simulink subsystem "PvtSubSys_LONC"  (R2020b)
settings: Solver=VariableStepAuto  StartTime=0.0  StopTime=10.0  RelTol=1e-3
undefined symbols (not defined in the file): P_Global_TireRadius_m, P_Global_Weight_N, P_LongCtrl_AxvRoadSlopeThrd, P_LongCtrl_SlideFlagEnable, P_LongCtrl_TotWheelTrqRatio, P_LongCtrl_VLC_fRollCoef, P_LongCtrl_VLC_WindArea, P_LongCtrl_VLCaccelMinHoldXAxis, P_LongCtrl_VLCaccelMinHoldYAxis, P_LongCtrl_VLCaccelMinSlidHoldXAxis, P_LongCtrl_VLCaccelMinSlidHoldYAxis, P_LongCtrl_VLCaDiffCharCoefKiEnableXAxis, P_LongCtrl_VLCaDiffCharCoefKiXAxis, P_LongCtrl_VLCaDtThresUpdateTorq, P_LongCtrl_VLCaXCDeadZoneProp_Y, P_LongCtrl_VLCaxCtrlDevDeadZoneChar_Y, P_LongCtrl_VLCaxCtrlDevEC2DCMax, P_LongCtrl_VLCaxCtrlDevFastQuitDCMode, P_LongCtrl_VLCaxCtrlDevThresAddEC2DCCharYAxis, P_LongCtrl_VLCaxCtrlDevTresAddDC2ECYAxis, P_LongCtrl_VLCaxDtCharAxCtrlDevTresAddDC2ECXAxis, P_LongCtrl_VLCaxDtCharAxCtrlDevTresAddEC2DCXAxis, P_LongCtrl_VLCAxTarDtThreEnableI, P_LongCtrl_VLCaxvRoadSlopeDC4CharXAxis, P_LongCtrl_VLCaxvRoadSlopeDC4CharYAxis, P_LongCtrl_VLCAxvTracMinDC1FullFillXAxis, P_LongCtrl_VLCAxvTracMinDC1FullFillYAxis, P_LongCtrl_VLCcoefFXAxis, P_LongCtrl_VLCcoefFYAxis, P_LongCtrl_VLCcoefIFadeOut1Calc, P_LongCtrl_VLCcoefIFadeOut1Condition, P_LongCtrl_VLCcoefIFadeOut2Calc, P_LongCtrl_VLCcoefIFadeOut2Condition, P_LongCtrl_VLCcoefIFadeOut3Calc, P_LongCtrl_VLCcoefIFadeOut3Condition, P_LongCtrl_VLCcoefKiDiffDtEnlargeYAxis, P_LongCtrl_VLCcoefKiEnableYAxis, P_LongCtrl_VLCcoefKiEnlargeADiffYAxis, P_LongCtrl_VLCcoefPIYAxis, P_LongCtrl_VLCCounterAxvTracMinTimeout, P_LongCtrl_VLCCounterDC2ECTorqDelay, P_LongCtrl_VLCCounterDrvOff2EC, P_LongCtrl_VLCdaxTarEC2DCMax, P_LongCtrl_VLCdiffDtCharCoefKiEnlargeXAxis, P_LongCtrl_VLCdriveOffAxUpLimXAxix, P_LongCtrl_VLCdriveOffAxUpLimYAxix, P_LongCtrl_VLCDtAxvRef2UpperBandDC5, P_LongCtrl_VLCengEfficientCharYAxis, P_LongCtrl_VLCengInverseEfficientYAxis, P_LongCtrl_VLCIACompensionNeg, P_LongCtrl_VLCIACompensionPos, P_LongCtrl_VLCjerkHoldXAxis, P_LongCtrl_VLCjerkHoldYAxis, P_LongCtrl_VLCjerkSlidHoldXAxis, P_LongCtrl_VLCjerkSlidHoldYAxis, P_LongCtrl_VLCki, P_LongCtrl_VLCkp, P_LongCtrl_VLCks, P_LongCtrl_VLCLowerJerkCounterDrvOff2EC, P_LongCtrl_VLCMaRatioCharMaYAxis ... (+12)
libraries: simulink x34
(part 3 of 3)

== matlab function PvtSubSys_LONC/VLC/Vlc/PI_Control/MATLAB Function ==
  data: I_k1 input single; Err input single; ECenable input boolean; I output single; Limited output single; axvFilt output single; Diff input single; tCycle input single; P_VlcWindupLim input single; AxTarDt input single; axv input single; tConst input single; VlcAxTar input single; ShiftInProgress input boolean; axvFiltK1 input single; P_LongCtrl_VLCAxTarDtThreEnableI parameter single; P_LongCtrl_VLCcoefIFadeOut1Condition parameter single; P_LongCtrl_VLCcoefIFadeOut1Calc parameter single; P_LongCtrl_VLCcoefIFadeOut2Condition parameter single; P_LongCtrl_VLCcoefIFadeOut2Calc parameter single; P_LongCtrl_VLCcoefIFadeOut3Condition parameter single; P_LongCtrl_VLCcoefIFadeOut3Calc parameter single; P_LongCtrl_VLCIACompensionPos parameter single; P_LongCtrl_VLCIACompensionNeg parameter single
function [I,Limited,axvFilt] = calcI(I_k1,Err,ECenable,Diff,tCycle,P_VlcWindupLim,AxTarDt,axv,tConst,VlcAxTar,ShiftInProgress,axvFiltK1,P_LongCtrl_VLCAxTarDtThreEnableI, P_LongCtrl_VLCcoefIFadeOut1Condition, P_LongCtrl_VLCcoefIFadeOut1Calc, P_LongCtrl_VLCcoefIFadeOut2Condition, P_LongCtrl_VLCcoefIFadeOut2Calc,...
      P_LongCtrl_VLCcoefIFadeOut3Condition, P_LongCtrl_VLCcoefIFadeOut3Calc, P_LongCtrl_VLCIACompensionPos, P_LongCtrl_VLCIACompensionNeg)
tau=tCycle/tConst;
axvFilt=tau*(axv-axvFiltK1)+axvFiltK1;
if ShiftInProgress==0
    if (((I_k1>0)&&(Diff>0))||((I_k1<=0)&&(Diff<=0)))&&(abs(AxTarDt)<P_LongCtrl_VLCAxTarDtThreEnableI)
         t_I =Diff*tCycle;   
    else
         if abs(Diff)>P_LongCtrl_VLCcoefIFadeOut1Condition*Err
             t_I =P_LongCtrl_VLCcoefIFadeOut1Calc*Diff*tCycle;
         elseif abs(Diff)>P_LongCtrl_VLCcoefIFadeOut2Condition*Err
                 t_I =P_LongCtrl_VLCcoefIFadeOut2Calc*Diff*tCycle;
             elseif abs(Diff)>P_LongCtrl_VLCcoefIFadeOut3Condition*Err
                     t_I =P_LongCtrl_VLCcoefIFadeOut3Calc*Diff*tCycle;
                 else 
                     t_I =Diff*tCycle;
         end       
    end
    if ((abs(AxTarDt)<P_LongCtrl_VLCAxTarDtThreEnableI)&&(abs(Diff)<Err))
         if (abs(VlcAxTar)>0.001&&(abs(axvFilt)<Err))
             if VlcAxTar>0.001
                Icompension=P_LongCtrl_VLCIACompensionPos*tCycle;
             else
                if VlcAxTar<-0.001
                   Icompension=P_LongCtrl_VLCIACompensionNeg*tCycle;
                else
                   Icompension=single(0);
                end
             end
         else
             Icompension=single(0);
         end
         if (abs(VlcAxTar)<0.001&&(abs(axvFilt)<Err))
              Istability=-axvFilt*tCycle;
         else
             Istability=single(0);
         end         
    else
      Icompension=single(0);
      Istability=single(0);
    end   
          t_I=I_k1+t_I+Icompension+Istability; 
          t_I =max(min(P_VlcWindupLim,t_I),-P_VlcWindupLim);
          if (t_I==P_VlcWindupLim)||(t_I==(-P_VlcWindupLim))
              Limited =single(1);
          else
              Limited =single(0);
          end
          if ECenable  
             I = t_I;
          else
             I = single(0);
          end
else
      I = single(0.5)*I_k1;
      Limited=single(0);
end

== matlab function PvtSubSys_LONC/VLC/Vlc/SwitchToBrakeMode/Switch ==
  data: AxTarEnable input boolean; y output boolean; DevEnable input boolean; BrakePrefer input boolean; ACC_Mode input uint8; StopReq input boolean; Sw1 input boolean; Sw2 input boolean; Sw3 input boolean; Sw4 input boolean; Sw5 input boolean; Sw6 input boolean; Sw7 input boolean
function y = fcn(AxTarEnable,DevEnable,BrakePrefer,ACC_Mode,StopReq,Sw1,Sw2,Sw3,Sw4,Sw5,Sw6,Sw7)
%#codegen

if (ACC_Mode==6)||(ACC_Mode==9)||(StopReq==1)
   y=true;
else
   if BrakePrefer
       y = Sw1;
   else
      if (AxTarEnable==1)||(DevEnable==1)
          y = Sw1&&Sw2&&Sw3&&Sw4&&Sw7; 
      else
          y = Sw1&&Sw2&&Sw3&&Sw4&&Sw5&&Sw6&&Sw7; 
      end
   end
end

== matlab function PvtSubSys_LONC/VLC/Vlc/SwitchToDriveMode/Switch ==
  data: Active input; y output; BrakePrefer input; StopReq input; Sw1 input; Sw2 input; Sw3 input; Sw4 input; Sw5 input; DriveOff2EC input
function y = fcn(Active,BrakePrefer,StopReq,Sw1,Sw2,Sw3,Sw4,Sw5,DriveOff2EC)
%#codegen
if Active
   if BrakePrefer||StopReq
       y=false;
   else
      if Sw5
          y = Sw1;
      else
          y = Sw1&&Sw2&&Sw3&&Sw4;
      end
   end
   if DriveOff2EC
       y=true;
   end
else
    y=false;
end

== matlab function PvtSubSys_LONC/VLC/Vlc/UpdateFlagCalc/Timer/MATLAB Function ==
  data: Falling input; Timer output single; StartTimer output single; TimerK1 input; StartTimerK1 input
function [Timer,StartTimer]= fcn(Falling,TimerK1,StartTimerK1)
StartTimer=StartTimerK1;
Timer=single(0);
if Falling==1
    StartTimer=single(1);
end
if StartTimer==1
    Timer=TimerK1+single(0.02);
end
if Timer>0.5
    StartTimer=single(0);
end

== stateflow chart PvtSubSys_LONC/VLC/Vlc/VLC_control_sts ==
  settings: executeAtInitialization=1
  state Init
  state Failure
  state Off
  state Active
    state DC
      entry:DCEnable=true;
      entry:tDC=1;
      during:tDC=min(tDC+1,200);
      exit:DCEnable=false;
      exit:tDC=0;
    state EC
      entry:ECEnable=true;
      entry:tEC=1;
      during:tEC=min(tEC+1,200);
      exit:ECEnable=false;
      exit:tEC=0;
    state Override
    state ECDC
      state ECDC2
        entry:VLCState = 3;
        entry:DCEnable=true;
        entry:ECEnable=true;
        entry:tECDC=1;
        during:tECDC=min(tECDC+1,200);
        exit:VLCState = 0;
        exit:DCEnable=false;
        exit:ECEnable=false;
        exit:tECDC=0;
      state ECDC1
        entry:VLCState = 3;
        entry:DCEnable=true;
        entry:ECEnable=false;
        exit:VLCState = 0;
        exit:DCEnable=false;
        exit:ECEnable=false;
      (default) -> ECDC1
      ECDC1 -> ECDC2 : [(SwitchToDriveMode==1)||...
          | (DriveOffConditonFulfilled)]
    (junction 85) -> DC [order 1] : [(ACC_Mode==6)||(ACC_Mode==9)]
    (junction 85) -> EC [order 2] : [(ACC_Mode!=6)&&(ACC_Mode!=9)]
    EC -> DC [order 2] : [SwitchToBrakeMode==1]
    DC -> EC [order 1] : [(SwitchToDriveMode==1)&&(tDC>=25*Motorial)]
    (junction 60) -> DC [order 2] : [OverrideToDC==1]
    (junction 60) -> EC [order 1] : [OverrideToDC==0]
    Override -> (junction 60) : [ACC_Mode~=5]
    DC -> ECDC [order 2] : [SlideFlag]
    DC -> (junction 91) [order 3]
    EC -> (junction 91) [order 3]
    EC -> ECDC [order 1] : [SlideFlag]
    ECDC -> EC [order 2] : [ForwardFlag]
    (junction 91) -> Override : [ACC_Mode==5]
    ECDC -> (junction 91) [order 1]
  (default) -> Init
  Failure -> Init : [VLCInternalFailSts==0]
  Init -> (junction 30)
  (junction 30) -> Failure [order 1] : [VLCInternalFailSts==1]
  (junction 30) -> Off [order 2] : [VLCInternalFailSts==0]
  (junction 39) -> Failure : [VLCInternalFailSts==1]
  Off -> (junction 39) [order 2]
  Active -> (junction 39) [order 1]
  Off -> (junction 85) [order 1] : [(ACC_Mode==3)||...
      | (ACC_Mode==6)||...
      | (ACC_Mode==5)||...
      | (ACC_Mode==9)]
  Active -> Off [order 2] : [(ACC_Mode==0)||...
      | (ACC_Mode==1)||...
      | (ACC_Mode==2)||...
      | (ACC_Mode==7)]
  data: SwitchToDriveMode input; SwitchToBrakeMode input; ECEnable output boolean; tEC output single; tDC output single; ACC_Mode input; DCEnable output boolean; VLCInternalFailSts input; Motorial input single; OverrideToDC input single; SlideFlag input; ForwardFlag input; DriveOffConditonFulfilled input; VLCState output double; tECDC output double

== matlab function PvtSubSys_LONC/VLC/Vlc/VlcInternalAccCalc ==
  data: EC input; DC input; DriveOff input; ACC_Mode input; VlcInternalAcc output single; AxRef input; AxTar input; AcceJerk input; DeceJerk input; DriveOffAxUpLim input; VlcInternalAccK1 input; tCycleVLC input
function VlcInternalAcc = CalcVlcInternalAcc(EC,DC,DriveOff,ACC_Mode,AxRef,AxTar,AcceJerk,DeceJerk,DriveOffAxUpLim,VlcInternalAccK1,tCycleVLC)
%#codegen
if ACC_Mode(1)==3
    if (DriveOff(1)==1)&&(DriveOff(2)==0)
           VlcInternalAcc = single(0.2);  
    else
       if ((VlcInternalAccK1>AxTar)&&(AxTar>=AxRef))||((VlcInternalAccK1<AxTar)&&(AxTar<=AxRef))
           VlcInternalAcc = AxTar;
       else
           if ((VlcInternalAccK1+DeceJerk*tCycleVLC)>AxRef)&&(AxRef>AxTar)
               VlcInternalAcc = AxRef+DeceJerk*tCycleVLC;
           else
               if ((VlcInternalAccK1+AcceJerk*tCycleVLC)<AxRef)&&(AxRef<AxTar)
                   VlcInternalAcc = AxRef+AcceJerk*tCycleVLC;
               else
                   VlcInternalAcc = max(min(AxTar,VlcInternalAccK1+AcceJerk*tCycleVLC),VlcInternalAccK1+DeceJerk*tCycleVLC);
               end
           end
       end
    end
else
   if ACC_Mode(1)==6||ACC_Mode(1)==9
%        VlcInternalAcc=single(0);
       VlcInternalAcc = max(min(AxTar,VlcInternalAccK1+AcceJerk*tCycleVLC),VlcInternalAccK1+DeceJerk*tCycleVLC);
   else
       VlcInternalAcc=AxRef;
   end
end
VlcInternalAcc = min(DriveOffAxUpLim,VlcInternalAcc);
